simulink model "RC3_EKF"  (R2025a)
settings: Solver=VariableStepAuto  StartTime=0.0  StopTime=length(Current)  RelTol=1e-3
values from neighbouring files (symbols this model uses):
  C1_est = [C1_est(1); C1_est]    [RC3_Parameter_Extract.m]
  C2_est = [C2_est(1); C2_est]    [RC3_Parameter_Extract.m]
  C3_est = [C3_est(1); C3_est]    [RC3_Parameter_Extract.m]
  OCV_fit = flipud(OCV_fit)    [RC3_Parameter_Extract.m]    (also in RC3_Parameter_Tuning.m)
  R0_est = [R0_est(1); R0_est]    [RC3_Parameter_Extract.m]
  R1_est = [R1_est(1); R1_est]    [RC3_Parameter_Extract.m]    (also in RC3_Parameter_Tuning.m = R1_est/10)
  R2_est = [R0_est(1); R2_est]    [RC3_Parameter_Extract.m]
  R3_est = [R3_est(1); R3_est]    [RC3_Parameter_Extract.m]
  SOC_OCV = [0:0.05:1]'    [RC3_Parameter_Extract.m]    (also in RC3_Parameter_Tuning.m)
  SOC_RC = [0:0.05:1]'    [RC3_Parameter_Extract.m]    (also in RC3_Parameter_Tuning.m = [0.05:0.05:1]')
settings Model: Creator=송민우  LastModifiedBy=Administrator

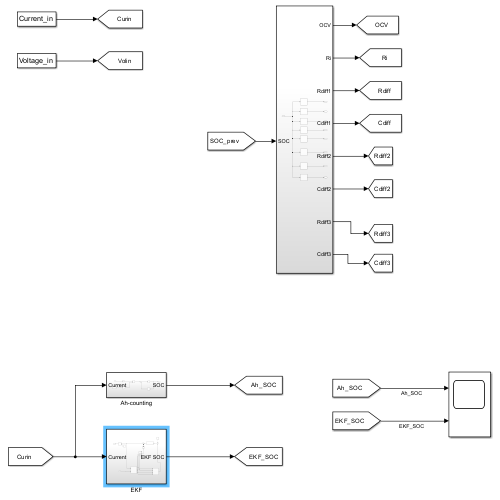
[thumbnail: Simulink's stored preview of the top-level diagram]
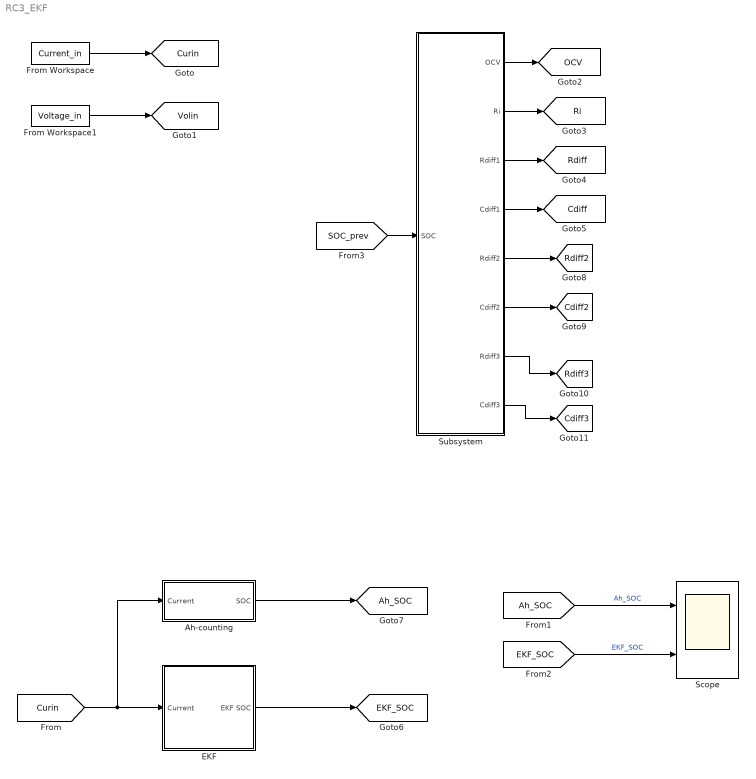
== system RC3_EKF ==
  Ah-counting : Subsystem
  EKF : Subsystem
  From Workspace : FromWorkspace  VariableName=Current_in  OutDataTypeStr=double  SampleTime=1
  From Workspace1 : FromWorkspace  VariableName=Voltage_in  OutDataTypeStr=double  SampleTime=1
  Scope : Scope  NumInputPorts=2
      settings: ActiveDisplayYMinimum=-0.12516694768269107  ActiveDisplayYMaximum=1.1255620860044682
  Subsystem : Subsystem
  tag scope: Ah_SOC=global, Cdiff2=global, Cdiff3=global, Cdiff=global, Curin=global, EKF_SOC=global, OCV=global, Rdiff2=global, Rdiff3=global, Rdiff=global, Ri=global, Volin=global
  wires:
  From Workspace/1 -> [Curin]
  From Workspace1/1 -> [Volin]
  [Curin] -> Ah-counting/1(Current), EKF/1(Current)
  [SOC_prev] -> Subsystem/1(SOC)
  Subsystem/1(OCV) -> [OCV]
  Subsystem/2(Ri) -> [Ri]
  Subsystem/3(Rdiff1) -> [Rdiff]
  Subsystem/4(Cdiff1) -> [Cdiff]
  EKF/1(EKF SOC) -> [EKF_SOC]
  Ah-counting/1(SOC) -> [Ah_SOC]
  [Ah_SOC] -> Scope/1  "Ah_SOC"
  [EKF_SOC] -> Scope/2  "EKF_SOC"
  Subsystem/5(Rdiff2) -> [Rdiff2]
  Subsystem/6(Cdiff2) -> [Cdiff2]
  Subsystem/7(Rdiff3) -> [Rdiff3]
  Subsystem/8(Cdiff3) -> [Cdiff3]

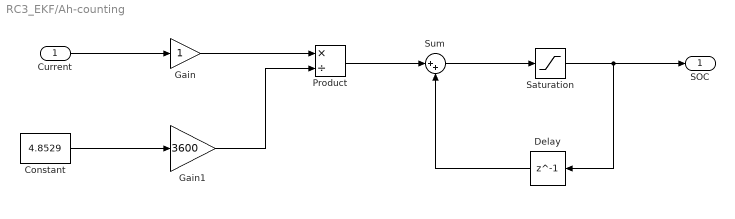
== system RC3_EKF/Ah-counting ==
  Current : Inport
  Constant : Constant  Value=4.8529
  Delay : Delay  DelayLength=1  InitialCondition=1
  Gain : Gain
  Gain1 : Gain  Gain=3600
  Product : Product  Inputs=*/
  Saturation : Saturate  UpperLimit=1  LowerLimit=0
  Sum : Sum  Inputs=|++
  SOC : Outport
  wires:
  Current/1 -> Gain/1
  Constant/1 -> Gain1/1
  Gain/1 -> Product/1
  Gain1/1 -> Product/2
  Product/1 -> Sum/1
  Sum/1 -> Saturation/1
  Saturation/1 -> Delay/1, SOC/1
  Delay/1 -> Sum/2

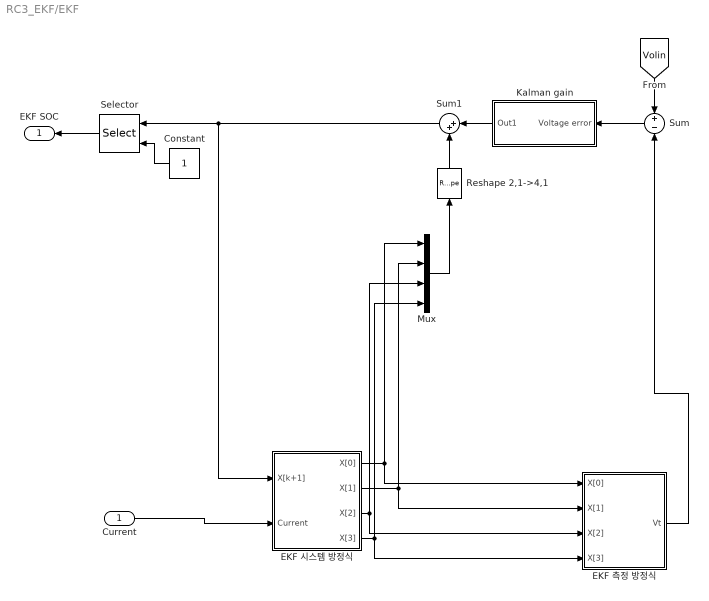
== system RC3_EKF/EKF ==
  Current : Inport
  Constant : Constant
  EKF 시스템 방정식 : Subsystem
  EKF 측정 방정식 : Subsystem
  Kalman gain : Subsystem
  Mux : Mux
  Reshape 2,1->4,1 : Reshape  OutputDimensionality=Customize  OutputDimensions=[4,1]
  Selector : Selector  InputPortWidth=4  IndexOptions=Index vector (port)  Indices=[1 3]  OutputSizes=1
  Sum : Sum  Inputs=+|-
  Sum1 : Sum  Inputs=|++
  EKF SOC : Outport
  wires:
  EKF 시스템 방정식/1(X[0]) -> Mux/1, EKF 측정 방정식/1(X[0])
  EKF 시스템 방정식/2(X[1]) -> Mux/2, EKF 측정 방정식/2(X[1])
  [Volin] -> Sum/1
  Sum/1 -> Kalman gain/1(Voltage error)
  Mux/1 -> Reshape 2,1->4,1/1
  Kalman gain/1(Out1) -> Sum1/1
  Reshape 2,1->4,1/1 -> Sum1/2
  Sum1/1 -> Selector/1, EKF 시스템 방정식/1(X[k+1])
  Current/1 -> EKF 시스템 방정식/2(Current)
  Constant/1 -> Selector/2
  Selector/1 -> EKF SOC/1
  EKF 시스템 방정식/3(X[2]) -> Mux/3, EKF 측정 방정식/3(X[2])
  EKF 시스템 방정식/4(X[3]) -> EKF 측정 방정식/4(X[3]), Mux/4
  EKF 측정 방정식/1(Vt) -> Sum/2

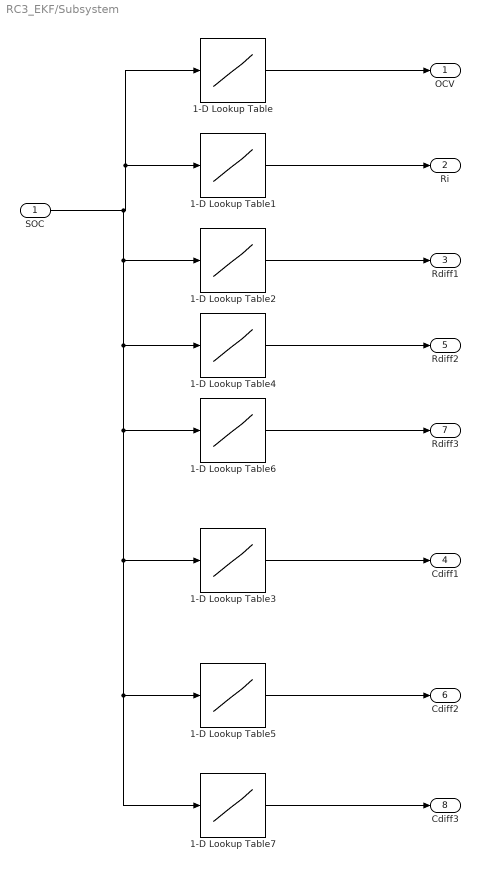
== system RC3_EKF/Subsystem ==
  SOC : Inport
  1-D Lookup Table : Lookup_n-D  NumberOfTableDimensions=1  BreakpointsForDimension1=SOC_OCV  Table=OCV_fit  InternalRulePriority=Speed  RndMeth=Simplest
  1-D Lookup Table1 : Lookup_n-D  NumberOfTableDimensions=1  BreakpointsForDimension1=SOC_RC  Table=R0_est  InternalRulePriority=Speed  RndMeth=Simplest
  1-D Lookup Table2 : Lookup_n-D  NumberOfTableDimensions=1  BreakpointsForDimension1=SOC_RC  Table=R1_est  InternalRulePriority=Speed  RndMeth=Simplest
  1-D Lookup Table3 : Lookup_n-D  NumberOfTableDimensions=1  BreakpointsForDimension1=SOC_RC  Table=C1_est  InternalRulePriority=Speed  RndMeth=Simplest
  1-D Lookup Table4 : Lookup_n-D  NumberOfTableDimensions=1  BreakpointsForDimension1=SOC_RC  Table=R2_est  InternalRulePriority=Speed  RndMeth=Simplest
  1-D Lookup Table5 : Lookup_n-D  NumberOfTableDimensions=1  BreakpointsForDimension1=SOC_RC  Table=C2_est  InternalRulePriority=Speed  RndMeth=Simplest
  1-D Lookup Table6 : Lookup_n-D  NumberOfTableDimensions=1  BreakpointsForDimension1=SOC_RC  Table=R3_est  InternalRulePriority=Speed  RndMeth=Simplest
  1-D Lookup Table7 : Lookup_n-D  NumberOfTableDimensions=1  BreakpointsForDimension1=SOC_RC  Table=C3_est  InternalRulePriority=Speed  RndMeth=Simplest
  OCV : Outport
  Ri : Outport  Port=2
  Rdiff1 : Outport  Port=3
  Cdiff1 : Outport  Port=4
  Rdiff2 : Outport  Port=5
  Cdiff2 : Outport  Port=6
  Rdiff3 : Outport  Port=7
  Cdiff3 : Outport  Port=8
  wires:
  1-D Lookup Table/1 -> OCV/1
  1-D Lookup Table1/1 -> Ri/1
  1-D Lookup Table3/1 -> Cdiff1/1
  1-D Lookup Table2/1 -> Rdiff1/1
  SOC/1 -> 1-D Lookup Table1/1, 1-D Lookup Table/1, 1-D Lookup Table4/1, 1-D Lookup Table6/1, 1-D Lookup Table3/1, 1-D Lookup Table5/1, 1-D Lookup Table7/1, 1-D Lookup Table2/1
  1-D Lookup Table7/1 -> Cdiff3/1
  1-D Lookup Table5/1 -> Cdiff2/1
  1-D Lookup Table4/1 -> Rdiff2/1
  1-D Lookup Table6/1 -> Rdiff3/1

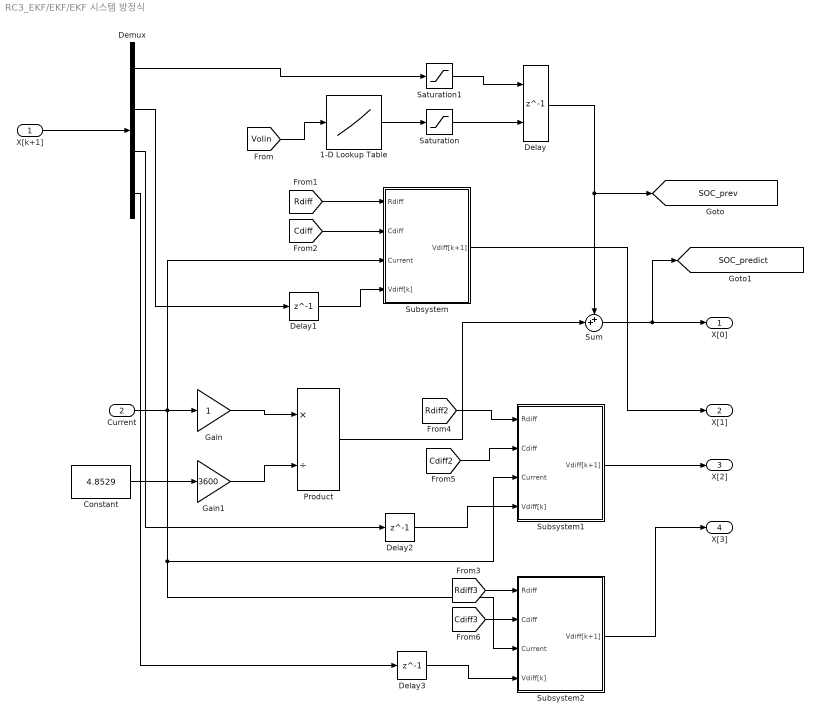
== system RC3_EKF/EKF/EKF 시스템 방정식 ==
  X[k+1] : Inport
  Current : Inport  Port=2
  1-D Lookup Table : Lookup_n-D  NumberOfTableDimensions=1  BreakpointsForDimension1=SOC_OCV  Table=OCV_fit  InternalRulePriority=Speed  RndMeth=Simplest
  Constant : Constant  Value=4.8529
  Delay : Delay  DelayLength=1  InitialConditionSource=Input port
      settings: InputPortMap=u0,p4
  Delay1 : Delay  DelayLength=1
  Delay2 : Delay  DelayLength=1
  Delay3 : Delay  DelayLength=1
  Demux : Demux
  Gain : Gain
  Gain1 : Gain  Gain=3600
  Product : Product  Inputs=*/
  Saturation : Saturate  UpperLimit=1  LowerLimit=0
  Saturation1 : Saturate  UpperLimit=1  LowerLimit=0
  Subsystem : Subsystem
  Subsystem1 : Subsystem
  Subsystem2 : Subsystem
  Sum : Sum  Inputs=++|
  X[0] : Outport
  X[1] : Outport  Port=2
  X[2] : Outport  Port=3
  X[3] : Outport  Port=4
  tag scope: SOC_predict=global, SOC_prev=global
  wires:
  X[k+1]/1 -> Demux/1
  [Volin] -> 1-D Lookup Table/1
  1-D Lookup Table/1 -> Saturation/1
  Saturation/1 -> Delay/2
  Saturation1/1 -> Delay/1
  Demux/1 -> Saturation1/1
  Current/1 -> Subsystem2/3(Current), Subsystem1/3(Current), Subsystem/3(Current), Gain/1
  Constant/1 -> Gain1/1
  Gain/1 -> Product/1
  Gain1/1 -> Product/2
  Product/1 -> Sum/2
  Delay/1 -> [SOC_prev], Sum/1
  Sum/1 -> [SOC_predict], X[0]/1
  [Rdiff] -> Subsystem/1(Rdiff)
  [Cdiff] -> Subsystem/2(Cdiff)
  Demux/2 -> Delay1/1
  Delay1/1 -> Subsystem/4(Vdiff[k])
  Subsystem/1(Vdiff[k+1]) -> X[1]/1
  Subsystem2/1(Vdiff[k+1]) -> X[3]/1
  Subsystem1/1(Vdiff[k+1]) -> X[2]/1
  Delay2/1 -> Subsystem1/4(Vdiff[k])
  Delay3/1 -> Subsystem2/4(Vdiff[k])
  Demux/3 -> Delay2/1
  Demux/4 -> Delay3/1
  [Rdiff2] -> Subsystem1/1(Rdiff)
  [Cdiff2] -> Subsystem1/2(Cdiff)
  [Rdiff3] -> Subsystem2/1(Rdiff)
  [Cdiff3] -> Subsystem2/2(Cdiff)

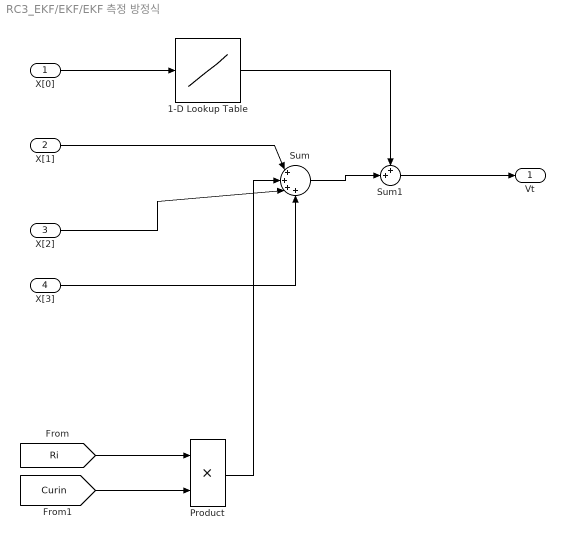
== system RC3_EKF/EKF/EKF 측정 방정식 ==
  X[0] : Inport
  X[1] : Inport  Port=2
  X[2] : Inport  Port=3
  X[3] : Inport  Port=4
  1-D Lookup Table : Lookup_n-D  NumberOfTableDimensions=1  BreakpointsForDimension1=SOC_OCV  Table=OCV_fit  InternalRulePriority=Speed  RndMeth=Simplest
  Product : Product
  Sum : Sum  Inputs=|++++
  Sum1 : Sum  Inputs=++|
  Vt : Outport
  wires:
  [Ri] -> Product/1
  [Curin] -> Product/2
  X[1]/1 -> Sum/1
  Product/1 -> Sum/2
  Sum/1 -> Sum1/2
  X[0]/1 -> 1-D Lookup Table/1
  1-D Lookup Table/1 -> Sum1/1
  Sum1/1 -> Vt/1
  X[2]/1 -> Sum/3
  X[3]/1 -> Sum/4

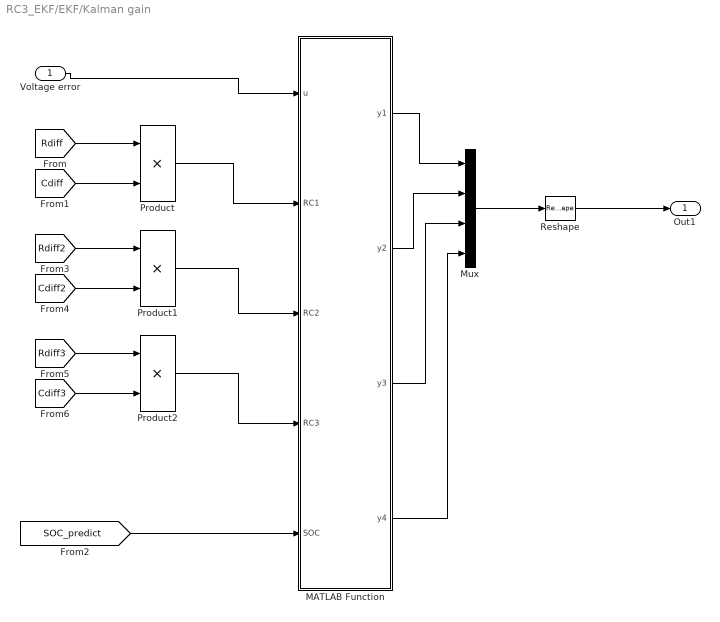
== system RC3_EKF/EKF/Kalman gain ==
  Voltage error : Inport
  MATLAB Function : MATLAB Function  TreatAsAtomicUnit=on
  Mux : Mux
  Product : Product
  Product1 : Product
  Product2 : Product
  Reshape : Reshape  OutputDimensionality=Customize  OutputDimensions=[4,1]
  Out1 : Outport
  wires:
  [Rdiff] -> Product/1
  [Cdiff] -> Product/2
  Voltage error/1 -> MATLAB Function/1(u)
  Product/1 -> MATLAB Function/2(RC1)
  [SOC_predict] -> MATLAB Function/5(SOC)
  MATLAB Function/1(y1) -> Mux/1
  MATLAB Function/2(y2) -> Mux/2
  Mux/1 -> Reshape/1
  Reshape/1 -> Out1/1
  Product1/1 -> MATLAB Function/3(RC2)
  [Rdiff2] -> Product1/1
  [Cdiff2] -> Product1/2
  [Cdiff3] -> Product2/2
  [Rdiff3] -> Product2/1
  Product2/1 -> MATLAB Function/4(RC3)
  MATLAB Function/3(y3) -> Mux/3
  MATLAB Function/4(y4) -> Mux/4

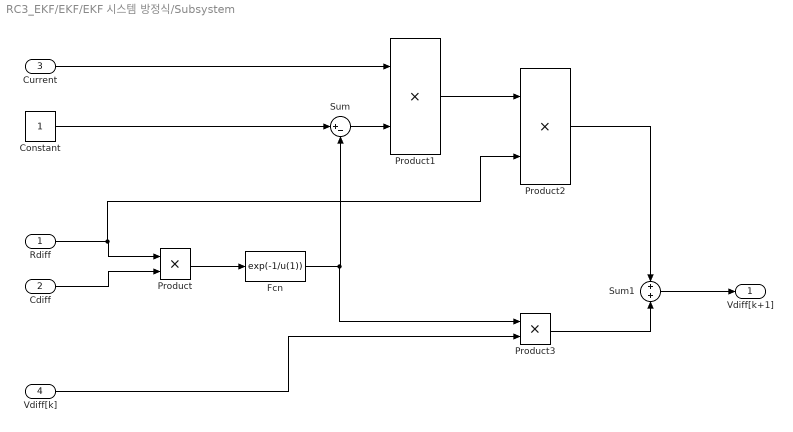
== system RC3_EKF/EKF/EKF 시스템 방정식/Subsystem ==
  Rdiff : Inport
  Cdiff : Inport  Port=2
  Current : Inport  Port=3
  Vdiff[k] : Inport  Port=4
  Constant : Constant
  Fcn : Fcn  Expr=exp(-1/u(1))
  Product{,1..3} (4 alike) : Product
  Sum : Sum  Inputs=|+-
  Sum1 : Sum  Inputs=+|+
  Vdiff[k+1] : Outport
  wires:
  Rdiff/1 -> Product2/2, Product/1
  Cdiff/1 -> Product/2
  Product/1 -> Fcn/1
  Constant/1 -> Sum/1
  Fcn/1 -> Product3/1, Sum/2
  Sum/1 -> Product1/2
  Current/1 -> Product1/1
  Product1/1 -> Product2/1
  Product2/1 -> Sum1/1
  Vdiff[k]/1 -> Product3/2
  Product3/1 -> Sum1/2
  Sum1/1 -> Vdiff[k+1]/1

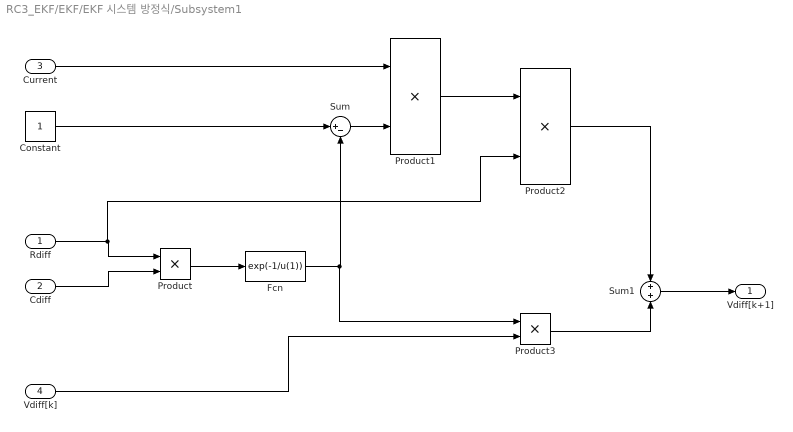
== system RC3_EKF/EKF/EKF 시스템 방정식/Subsystem1 ==
  Rdiff : Inport
  Cdiff : Inport  Port=2
  Current : Inport  Port=3
  Vdiff[k] : Inport  Port=4
  Constant : Constant
  Fcn : Fcn  Expr=exp(-1/u(1))
  Product{,1..3} (4 alike) : Product
  Sum : Sum  Inputs=|+-
  Sum1 : Sum  Inputs=+|+
  Vdiff[k+1] : Outport
  wires:
  Rdiff/1 -> Product2/2, Product/1
  Cdiff/1 -> Product/2
  Product/1 -> Fcn/1
  Constant/1 -> Sum/1
  Fcn/1 -> Product3/1, Sum/2
  Sum/1 -> Product1/2
  Current/1 -> Product1/1
  Product1/1 -> Product2/1
  Product2/1 -> Sum1/1
  Vdiff[k]/1 -> Product3/2
  Product3/1 -> Sum1/2
  Sum1/1 -> Vdiff[k+1]/1

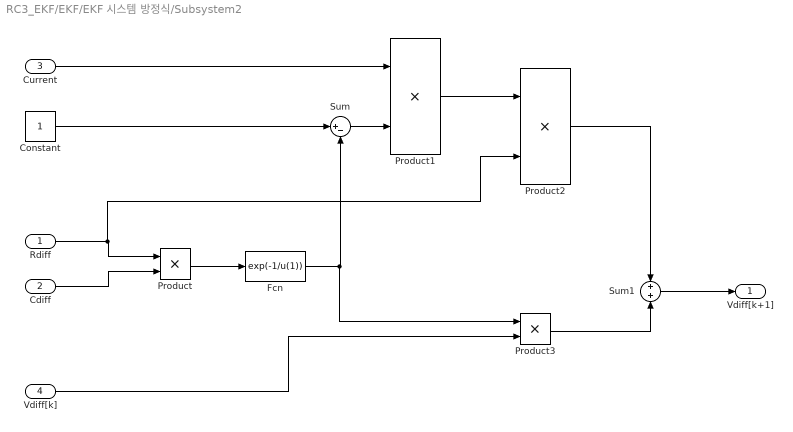
== system RC3_EKF/EKF/EKF 시스템 방정식/Subsystem2 ==
  Rdiff : Inport
  Cdiff : Inport  Port=2
  Current : Inport  Port=3
  Vdiff[k] : Inport  Port=4
  Constant : Constant
  Fcn : Fcn  Expr=exp(-1/u(1))
  Product{,1..3} (4 alike) : Product
  Sum : Sum  Inputs=|+-
  Sum1 : Sum  Inputs=+|+
  Vdiff[k+1] : Outport
  wires:
  Rdiff/1 -> Product2/2, Product/1
  Cdiff/1 -> Product/2
  Product/1 -> Fcn/1
  Constant/1 -> Sum/1
  Fcn/1 -> Product3/1, Sum/2
  Sum/1 -> Product1/2
  Current/1 -> Product1/1
  Product1/1 -> Product2/1
  Product2/1 -> Sum1/1
  Vdiff[k]/1 -> Product3/2
  Product3/1 -> Sum1/2
  Sum1/1 -> Vdiff[k+1]/1

== matlab function RC3_EKF/EKF/Kalman gain/MATLAB Function ==
  data: u input; y1 output; RC1 input; RC2 input; RC3 input; SOC input; y2 output; y3 output; y4 output
function [y1, y2,y3,y4] = fcn(u, RC1, RC2, RC3, SOC)

persistent P firstRun

dt=1;

    p1 = 221.4;
    p2 = -1154;
    p3 = 2509;
    p4 = -2932;
    p5 = 1981;
    p6 = -774;
    p7 = 167.4;
    p8 = -18.83;
    p9 = 1.644;

    H = [9*p1*SOC^8+8*p2*SOC^7+7*p3*SOC^6+6*p4*SOC^5+...
        5*p5*SOC^4+4*p6*SOC^3+3*p7*SOC^2+2*p8*SOC^1+p9 1 1 1];

    A = [1 0 0 0; 0 exp(-(dt/RC1)) 0 0; 0 0 exp(-(dt/RC2)) 0; 0 0 0 exp(-(dt/RC3))];
    Q = [0.0001 0 0 0;0 0.00001 0 0; 0 0 0.00001 0; 0 0 0 0.00001];
    R = 1e2;

if isempty(firstRun)

    P=[1 0 0 0;0 0 0 0;0 0 0 0;0 0 0 0];

    firstRun = 1;
end

Pp=A*P*A'+Q;

K=Pp*H'*inv(H*Pp*H'+R);

P=Pp-K*H*Pp;

y1=K(1)*u(1);
y2=K(2)*u(1);
y3=K(3)*u(1);
y4=K(4)*u(1);
